simulink model "UAV6DOF_Sim_Brian"  (R2024a)
settings: Solver=ode45  StartTime=0.0  StopTime=10  FixedStep=0.05  RelTol=1e-3  EnableMultiTasking=on
undefined symbols (not defined in the file or in its folder): alate, along, blate, blong, clate, clong, dlate, dlong, ytrim
settings Model: Creator=Administrator  LastModifiedBy=rzxha
settings SolverCC: AlgebraicLoopSolver=TrustRegion
settings DataIOCC: LimitDataPoints=on  SaveFormat=Array  SignalLoggingSaveFormat=ModelDataLogs  ReturnWorkspaceOutputs=off
settings OptimizationCC: ExpressionDepthLimit=2147483647  InitFltsAndDblsToZero=on  LifeSpan=inf
settings DebuggingCC: UnderspecifiedInitializationDetection=Classic  MergeDetectMultiDrivingBlocksExec=none  SolverPrmCheckMsg=warning  FcnCallInpInsideContextMsg=warning  UnconnectedInputMsg=warning  UnconnectedOutputMsg=warning  UnconnectedLineMsg=warning  StateNameClashWarn=warning  SFUnexpectedBacktrackingDiag=warning  SFNoUnconditionalDefaultTransitionDiag=warning  SFExecutionAtInitializationDiag=none  ArithmeticOperatorsInVariantConditions=warning
settings HardwareCC: ProdBitPerPointer=32  ProdBitPerSizeT=32  ProdBitPerPtrDiffT=32  ProdLargestAtomicFloat=None  ProdIntDivRoundTo=Undefined  ProdEndianess=Unspecified  ProdWordSize=32  ProdHWDeviceType=32-bit Generic
settings ModelReferenceCC: EnableRefExpFcnMdlSchedulingChecks=on  PropagateSignalLabelsOutOfModel=off
settings SFSimCC: SimUseLocalCustomCode=off  CustomCodeUndefinedFunction=UseInterfaceOnly
settings RTWCC: RTWUseLocalCustomCode=off  GPUComputeCapability=3.5
settings CodeAppCC: StateflowObjectComments=on
settings GRTTargetCC: TargetLangStandard=C89/C90 (ANSI)  CombineOutputUpdateFcns=off  GRTInterface=on
settings ConfigComp: CovMetricSettings=dw  CovSaveCumulativeToWorkspaceVar=on  CovSaveSingleToWorkspaceVar=on  CovExternalEMLEnable=off

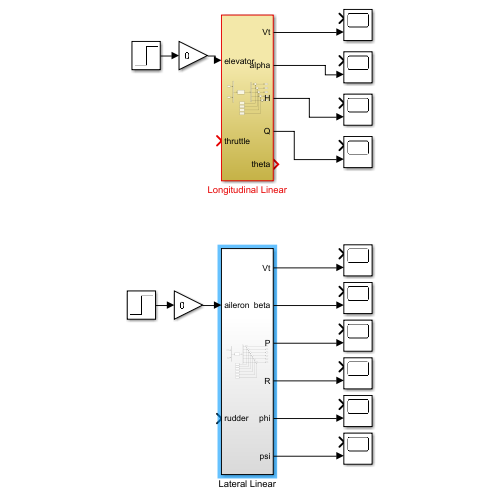
[thumbnail: Simulink's stored preview of the top-level diagram]
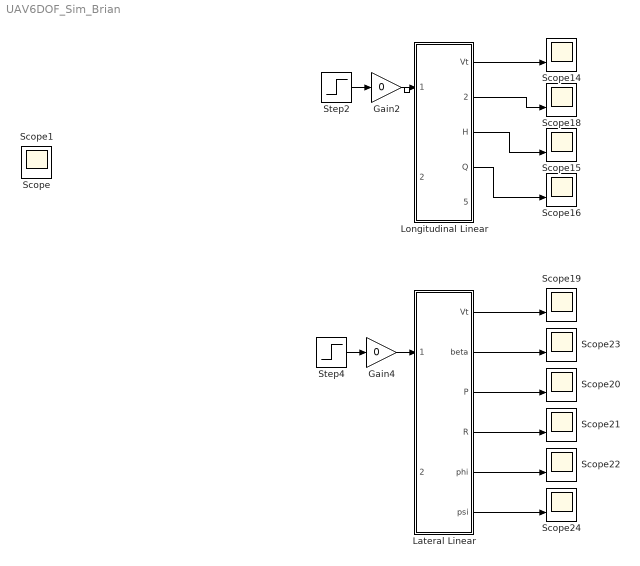
== system UAV6DOF_Sim_Brian ==
  Gain2 : Gain  Gain=0
  Gain4 : Gain  Gain=0
  Lateral Linear : Subsystem
  Longitudinal Linear : Subsystem
  Scope{14..16,18..24} (10 alike) : Scope  NumInputPorts=2
  Step2 : Step  SampleTime=0
  Step4 : Step  SampleTime=0
  Scope : Scope
  Scope1 : Scope
  wires:
  Step2/1 -> Gain2/1
  Step4/1 -> Gain4/1
  Gain2/1 -> Longitudinal Linear/1(elevator)
  Longitudinal Linear/1(Vt) -> Scope14/2
  Longitudinal Linear/3(H) -> Scope15/2
  Longitudinal Linear/4(Q) -> Scope16/2
  Gain4/1 -> Lateral Linear/1(aileron)
  Lateral Linear/1(Vt) -> Scope19/2
  Lateral Linear/2(beta) -> Scope23/2
  Lateral Linear/3(P) -> Scope20/2
  Lateral Linear/4(R) -> Scope21/2
  Lateral Linear/5(phi) -> Scope22/2
  Lateral Linear/6(psi) -> Scope24/2
  Longitudinal Linear/2(alpha) -> Scope18/2

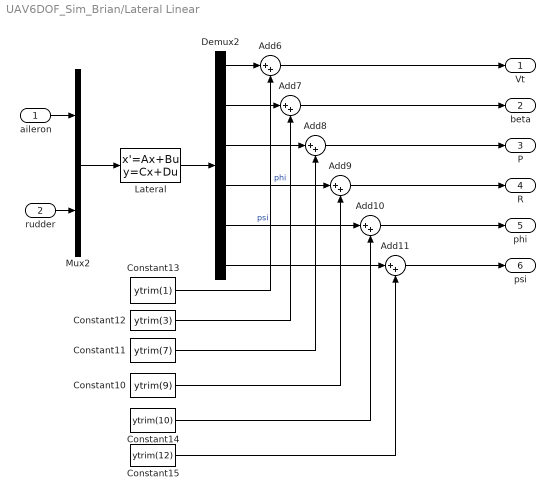
== system UAV6DOF_Sim_Brian/Lateral Linear ==
  aileron : Inport
  rudder : Inport  Port=2
  Add{6..11} (6 alike) : Sum  Inputs=|++
  Constant10 : Constant  Value=ytrim(9)
  Constant11 : Constant  Value=ytrim(7)
  Constant12 : Constant  Value=ytrim(3)
  Constant13 : Constant  Value=ytrim(1)
  Constant14 : Constant  Value=ytrim(10)
  Constant15 : Constant  Value=ytrim(12)
  Demux2 : Demux  Outputs=6
  Lateral : StateSpace  A=alate  B=blate  C=clate  D=dlate  InitialCondition=[0 deg2rad(1) 0 0 deg2rad(0) deg2rad(1)]
  Mux2 : Mux  Inputs=2
  Vt : Outport
  beta : Outport  Port=2
  P : Outport  Port=3
  R : Outport  Port=4
  phi : Outport  Port=5
  psi : Outport  Port=6
  wires:
  Constant12/1 -> Add7/2
  Demux2/4 -> Add9/1  "phi"
  Constant15/1 -> Add11/2
  Constant11/1 -> Add8/2
  Constant14/1 -> Add10/2
  Demux2/3 -> Add8/1
  Lateral/1 -> Demux2/1
  Demux2/5 -> Add10/1  "psi"
  aileron/1 -> Mux2/1
  Demux2/2 -> Add7/1
  rudder/1 -> Mux2/2
  Constant10/1 -> Add9/2
  Mux2/1 -> Lateral/1
  Demux2/6 -> Add11/1
  Demux2/1 -> Add6/1
  Constant13/1 -> Add6/2
  Add10/1 -> phi/1
  Add9/1 -> R/1
  Add6/1 -> Vt/1
  Add8/1 -> P/1
  Add7/1 -> beta/1
  Add11/1 -> psi/1

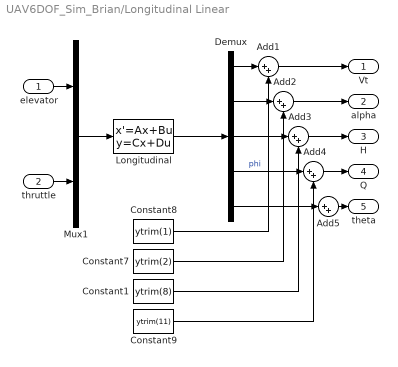
== system UAV6DOF_Sim_Brian/Longitudinal Linear ==
  elevator : Inport
  thruttle : Inport  Port=2
  Add{1..5} (5 alike) : Sum  Inputs=|++
  Constant1 : Constant  Value=ytrim(8)
  Constant7 : Constant  Value=ytrim(2)
  Constant8 : Constant  Value=ytrim(1)
  Constant9 : Constant  Value=ytrim(11)
  Demux : Demux  Outputs=5
  "Longitudinal " : StateSpace  A=along  B=blong  C=clong  D=dlong  InitialCondition=[0 deg2rad(1) 0 0 deg2rad(1)]
  Mux1 : Mux  Inputs=2
  Vt : Outport
  alpha : Outport  Port=2
  H : Outport  Port=3
  Q : Outport  Port=4
  theta : Outport  Port=5
  wires:
  Demux/2 -> Add2/1
  Demux/1 -> Add1/1
  Demux/3 -> Add3/1
  Constant1/1 -> Add3/2
  Mux1/1 -> "Longitudinal "/1
  Constant9/1 -> Add4/2
  Demux/4 -> Add4/1  "phi"
  Constant7/1 -> Add2/2
  Constant8/1 -> Add1/2
  "Longitudinal "/1 -> Demux/1
  thruttle/1 -> Mux1/2
  Add2/1 -> alpha/1
  Add3/1 -> H/1
  Add4/1 -> Q/1
  Add1/1 -> Vt/1
  elevator/1 -> Mux1/1
  Demux/5 -> Add5/1
  Add5/1 -> theta/1
